simulink model "AdvancedControlSim"  (R2021a)
settings: Solver=ode4  StartTime=0.0  StopTime=5  FixedStep=0.002  RelTol=1e-3
undefined symbols (not defined in the file or in its folder): A, Ap, B, Bp, C, ControllerIndex, D, gaussian, H2_inv_T, QNp, use_noise
libraries: simulink x3
settings Model: Creator=alexj  LastModifiedBy=alexj
settings SolverCC: AlgebraicLoopSolver=TrustRegion
settings DataIOCC: ReturnWorkspaceOutputs=off
settings DebuggingCC: SFMachineParentedDataDiag=warning  ArithmeticOperatorsInVariantConditions=warning
settings SFSimCC: CustomCodeUndefinedFunction=UseInterfaceOnly

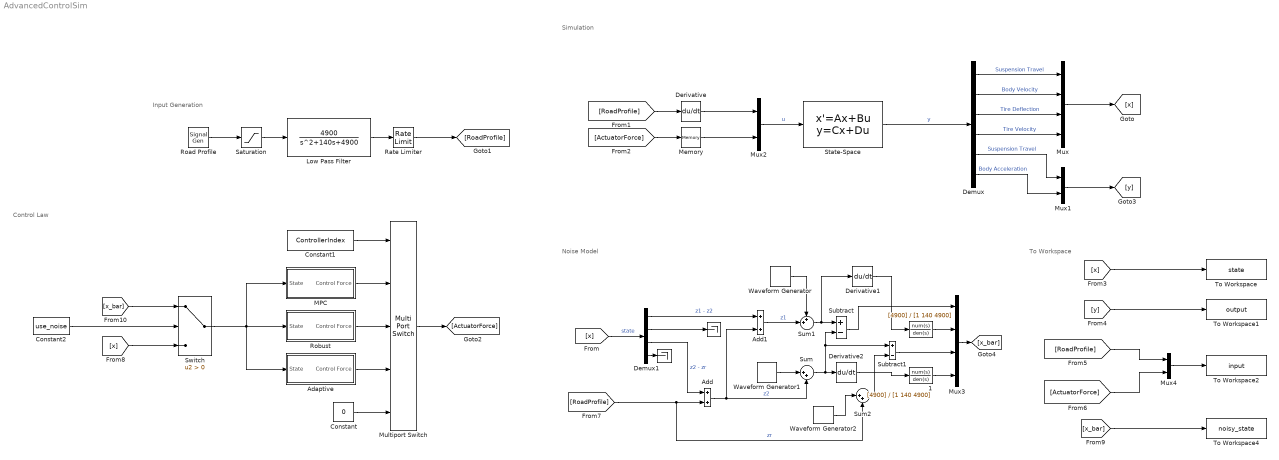
== system AdvancedControlSim ==
  note: Control Law
  note: To Workspace
  note: Noise Model
  note: Simulation
  note: Input Generation
  " " : Terminator
  "  " : Terminator
  "   " : TransferFcn  Numerator=[4900]  Denominator=[1 140 4900]
  "   1" : TransferFcn  Numerator=[4900]  Denominator=[1 140 4900]
  Adaptive : Subsystem
  Add : Sum
  Add1 : Sum
  Constant : Constant  Value=0
  Constant1 : Constant  Value=ControllerIndex
  Constant2 : Constant  Value=use_noise
  Demux : Demux  Outputs=6
  Demux1 : Demux
  Derivative : Derivative
  Derivative1 : Derivative
  Derivative2 : Derivative
  "Low Pass Filter " : TransferFcn  Numerator=[4900]  Denominator=[1 140 4900]
  MPC : Subsystem
  Memory : Memory
  Multiport Switch : MultiPortSwitch  DataPortForDefault=Additional data port  DiagnosticForDefault=None
  Mux : Mux
  Mux1 : Mux  Inputs=2
  Mux2 : Mux  Inputs=2
  Mux3 : Mux
  Mux4 : Mux  Inputs=2
  Rate Limiter : RateLimiter  RisingSlewLimit=0.2  FallingSlewLimit=-0.2  SampleTimeMode=inherited
  "Road Profile " : SignalGenerator  WaveForm=square  Amplitude=0.01  Frequency=0.3
  Robust : Subsystem
  Saturation : Saturate  UpperLimit=1  LowerLimit=-1
  State-Space : StateSpace  A=A  B=B  C=[eye(4);C]  D=[zeros(4,2);D]  InitialCondition=[0;0;0;0]
  Subtract : Sum  Inputs=+-
  Subtract1 : Sum  Inputs=+-
  Sum : Sum  Inputs=|++
  Sum1 : Sum  Inputs=++|
  Sum2 : Sum  Inputs=|++
  Switch : Switch  Criteria=u2 > Threshold
  To Workspace : ToWorkspace  VariableName=state  SaveFormat=Timeseries  SampleTime=-1
  To Workspace1 : ToWorkspace  VariableName=output  SaveFormat=Timeseries  SampleTime=-1
  To Workspace2 : ToWorkspace  VariableName=input  SaveFormat=Timeseries  SampleTime=-1
  To Workspace4 : ToWorkspace  VariableName=noisy_state  SaveFormat=Timeseries  SampleTime=-1
  Waveform Generator : simulink/Sources/Waveform Generator  OutMin=[]  OutMax=[]  OutDataTypeStr=double  SelectedSignal=1  Signals=gaussian('Mean', 0, 'Variance',5e-8,'Seed',31415)  BlockNames=MultiportSwitch_31f117a6580d47f  SampleTime=0.01
  Waveform Generator1 : simulink/Sources/Waveform Generator  OutMin=[]  OutMax=[]  OutDataTypeStr=double  SelectedSignal=1  Signals=gaussian('Mean', 0, 'Variance',5e-8,'Seed',17724)  BlockNames=MultiportSwitch_13f20ef5f3264e3  SampleTime=0.01
  Waveform Generator2 : simulink/Sources/Waveform Generator  OutMin=[]  OutMax=[]  OutDataTypeStr=double  SelectedSignal=1  Signals=gaussian('Mean', 0, 'Variance',5e-8,'Seed',9869)  BlockNames=MultiportSwitch_35dde4a2a30f460  SampleTime=0.01
  wires:
  Mux2/1 -> State-Space/1  "u"
  State-Space/1 -> Demux/1  "y"
  Demux/1 -> Mux/1  "Suspension Travel"
  Demux/2 -> Mux/2  "Body Velocity"
  Demux/3 -> Mux/3  "Tire Deflection"
  Demux/4 -> Mux/4  "Tire Velocity"
  Demux/6 -> Mux1/2  "Body Acceleration"
  Demux/5 -> Mux1/1  "Suspension Travel"
  Mux/1 -> [x]
  "Road Profile "/1 -> Saturation/1
  Saturation/1 -> "Low Pass Filter "/1
  "Low Pass Filter "/1 -> Rate Limiter/1
  Rate Limiter/1 -> [RoadProfile]
  [x] -> Demux1/1  "state"
  [RoadProfile] -> Derivative/1
  Derivative/1 -> Mux2/1
  Mux1/1 -> [y]
  [y] -> To Workspace1/1
  [x] -> To Workspace/1
  [RoadProfile] -> Add/2, Sum2/2  "zr"
  Demux1/3 -> Add/1  "z2 - zr"
  Demux1/4 -> " "/1
  Demux1/2 -> "  "/1
  Add/1 -> Sum/2, Add1/2  "z2"
  Demux1/1 -> Add1/1  "z1 - z2"
  Add1/1 -> Sum1/2  "z1"
  Sum1/1 -> Derivative1/1, Subtract/1
  Sum/1 -> Subtract/2, Subtract1/1, Derivative2/1
  Subtract/1 -> Mux3/1
  Sum2/1 -> Subtract1/2
  Subtract1/1 -> Mux3/3
  Mux3/1 -> [x_bar]
  [x_bar] -> To Workspace4/1
  [RoadProfile] -> Mux4/1
  [ActuatorForce] -> Mux4/2
  Mux4/1 -> To Workspace2/1
  "   "/1 -> Mux3/2
  "   1"/1 -> Mux3/4
  Waveform Generator2/1 -> Sum2/1
  Waveform Generator/1 -> Sum1/1
  Waveform Generator1/1 -> Sum/1
  Derivative1/1 -> "   "/1
  Derivative2/1 -> "   1"/1
  Robust/1(Control Force) -> Multiport Switch/3
  MPC/1(Control Force) -> Multiport Switch/2
  Adaptive/1(Control Force) -> Multiport Switch/4
  Constant/1 -> Multiport Switch/5
  Constant1/1 -> Multiport Switch/1
  Switch/1 -> MPC/1(State), Adaptive/1(State), Robust/1(State)
  [x] -> Switch/3
  [x_bar] -> Switch/1
  Constant2/1 -> Switch/2
  [ActuatorForce] -> Memory/1
  Memory/1 -> Mux2/2
  Multiport Switch/1 -> [ActuatorForce]

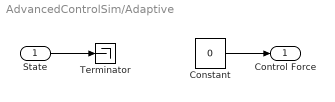
== system AdvancedControlSim/Adaptive ==
  State : Inport
  Constant : Constant  Value=0
  Terminator : Terminator
  Control Force : Outport
  wires:
  State/1 -> Terminator/1
  Constant/1 -> Control Force/1

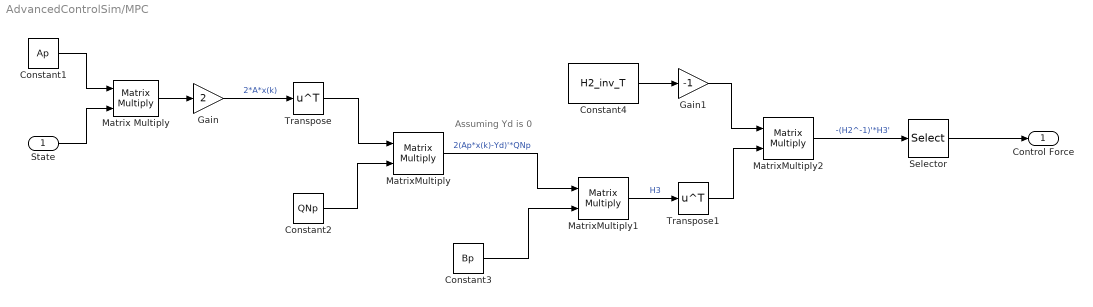
== system AdvancedControlSim/MPC ==
  note: Assuming Yd is 0
  State : Inport
  Constant1 : Constant  Value=Ap
  Constant2 : Constant  Value=QNp
  Constant3 : Constant  Value=Bp
  Constant4 : Constant  Value=H2_inv_T
  Gain : Gain  Gain=2
  Gain1 : Gain  Gain=-1
  Matrix Multiply : Product  Multiplication=Matrix(*)
  MatrixMultiply : Product  Multiplication=Matrix(*)
  MatrixMultiply1 : Product  Multiplication=Matrix(*)
  MatrixMultiply2 : Product  Multiplication=Matrix(*)
  Selector : Selector  InputPortWidth=Nc  IndexOptions=Index vector (dialog)  Indices=[1]  OutputSizes=1
  Transpose : Math  Operator=transpose  SaturateOnIntegerOverflow=on
  Transpose1 : Math  Operator=transpose  SaturateOnIntegerOverflow=on
  Control Force : Outport
  wires:
  State/1 -> Matrix Multiply/2
  Constant1/1 -> Matrix Multiply/1
  Matrix Multiply/1 -> Gain/1
  Gain/1 -> Transpose/1  "2*A*x(k)"
  Transpose/1 -> MatrixMultiply/1
  Constant2/1 -> MatrixMultiply/2
  MatrixMultiply/1 -> MatrixMultiply1/1  "2(Ap*x(k)-Yd)'*QNp"
  Constant3/1 -> MatrixMultiply1/2
  MatrixMultiply1/1 -> Transpose1/1  "H3"
  Constant4/1 -> Gain1/1
  Gain1/1 -> MatrixMultiply2/1
  Transpose1/1 -> MatrixMultiply2/2
  MatrixMultiply2/1 -> Selector/1  "-(H2^-1)'*H3'"
  Selector/1 -> Control Force/1

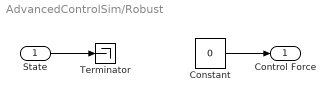
== system AdvancedControlSim/Robust ==
  State : Inport
  Constant : Constant  Value=0
  Terminator : Terminator
  Control Force : Outport
  wires:
  State/1 -> Terminator/1
  Constant/1 -> Control Force/1
